simulink model "motorQuantized"  (R2021b)
settings: Solver=VariableStepAuto  StartTime=0.0  StopTime=10.0  RelTol=1e-3
values from neighbouring files (symbols this model uses):
  b = 0.5    [Assignment2_Curtis.m]    (also in Assignment2m_Curtis.m)
  J = 0.05    [Assignment2_Curtis.m]    (also in Assignment2m_Curtis.m)
  Ke = 0.5    [Assignment2_Curtis.m]    (also in Assignment2m_Curtis.m)
  Kt = 0.5    [Assignment2_Curtis.m]    (also in Assignment2m_Curtis.m)
  Ra = 1    [Assignment2_Curtis.m]    (also in Assignment2m_Curtis.m)
settings Model: Creator=Alex  LastModifiedBy=Alex

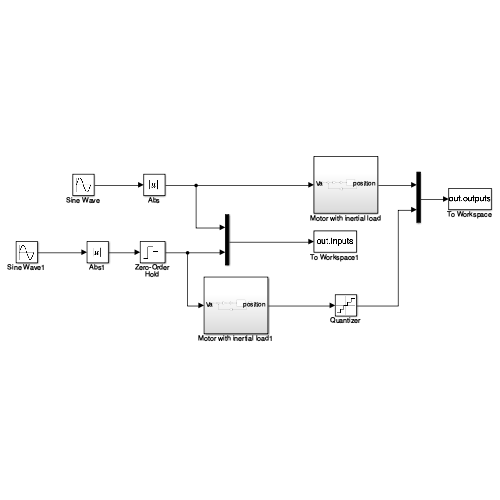
[thumbnail: Simulink's stored preview of the top-level diagram]
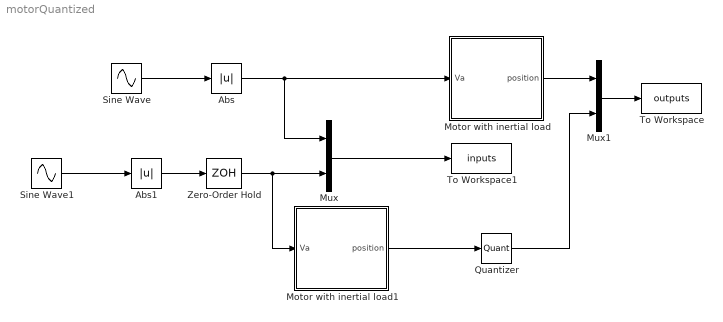
== system motorQuantized ==
  Abs : Abs
  Abs1 : Abs
  Motor with inertial load : Subsystem
  Motor with inertial load1 : Subsystem
  Mux : Mux  Inputs=2
  Mux1 : Mux  Inputs=2
  Quantizer : Quantizer
  Sine Wave : Sin  SampleTime=0
  Sine Wave1 : Sin  SampleTime=0
  To Workspace : ToWorkspace  VariableName=outputs  SaveFormat=Timeseries  SampleTime=-1
  To Workspace1 : ToWorkspace  VariableName=inputs  SaveFormat=Timeseries  SampleTime=-1
  Zero-Order Hold : ZeroOrderHold  SampleTime=-1
  wires:
  Abs/1 -> Mux/1, Motor with inertial load/1(Va)
  Zero-Order Hold/1 -> Mux/2, Motor with inertial load1/1(Va)
  Sine Wave/1 -> Abs/1
  Motor with inertial load/1(position) -> Mux1/1
  Abs1/1 -> Zero-Order Hold/1
  Motor with inertial load1/1(position) -> Quantizer/1
  Sine Wave1/1 -> Abs1/1
  Quantizer/1 -> Mux1/2
  Mux/1 -> To Workspace1/1
  Mux1/1 -> To Workspace/1

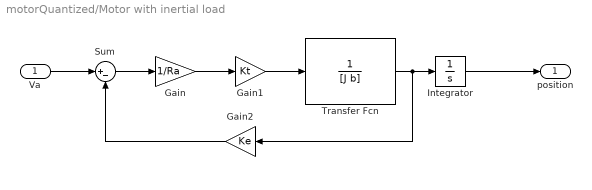
== system motorQuantized/Motor with inertial load ==
  Va : Inport
  Gain : Gain  Gain=1/Ra
  Gain1 : Gain  Gain=Kt
  Gain2 : Gain  Gain=Ke
  Integrator : Integrator
  Sum : Sum  Inputs=|+-
  Transfer Fcn : TransferFcn  Denominator=[J b]
  position : Outport
  wires:
  Va/1 -> Sum/1
  Integrator/1 -> position/1
  Sum/1 -> Gain/1
  Gain/1 -> Gain1/1
  Gain2/1 -> Sum/2
  Transfer Fcn/1 -> Integrator/1, Gain2/1
  Gain1/1 -> Transfer Fcn/1

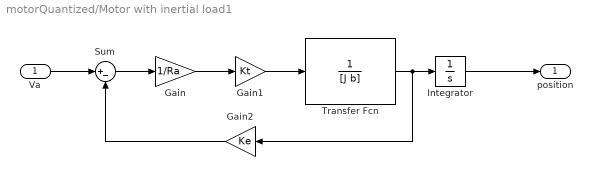
== system motorQuantized/Motor with inertial load1 ==
  Va : Inport
  Gain : Gain  Gain=1/Ra
  Gain1 : Gain  Gain=Kt
  Gain2 : Gain  Gain=Ke
  Integrator : Integrator
  Sum : Sum  Inputs=|+-
  Transfer Fcn : TransferFcn  Denominator=[J b]
  position : Outport
  wires:
  Va/1 -> Sum/1
  Integrator/1 -> position/1
  Sum/1 -> Gain/1
  Gain/1 -> Gain1/1
  Gain2/1 -> Sum/2
  Transfer Fcn/1 -> Integrator/1, Gain2/1
  Gain1/1 -> Transfer Fcn/1
